simulink model "opdracht1"  (Simulink 6.6)
settings: Solver=ode45  StartTime=0.0  StopTime=inf  RelTol=1e-3
libraries: dspsrcs4 x1, simulink x1, simulink_extras x1
settings Model: Creator=student  LastModifiedBy=student

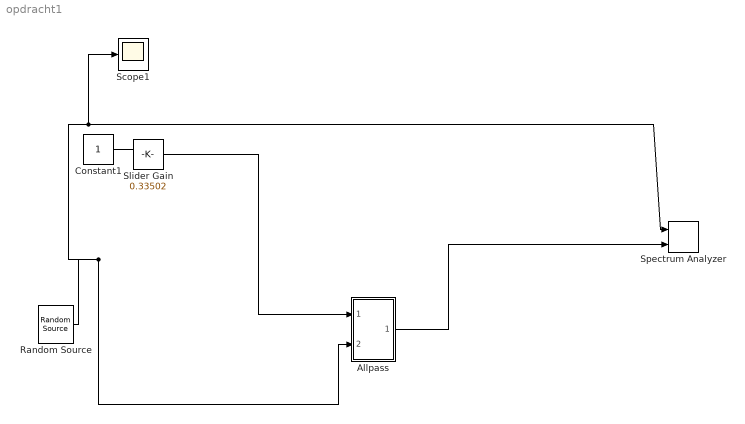
== system opdracht1 ==
  Allpass : Subsystem
  Constant1 : Constant
  Random Source : dspsrcs4/Random Source  SrcType=Uniform  NormMethod=Ziggurat  CltLength=12  MinVal=-10  MaxVal=10  MeanVal=0  VarVal=1  RepMode=Not repeatable  rawSeed=1  IsInherit=off  SampMode=Discrete  SampTime=1  SampFrame=1  DataType=Double  OutComplex=Real
  Scope1 : Scope
  Slider Gain : simulink/Math Operations/Slider Gain  SystemSampleTime=-1  low=0  gain=0.33502  high=1
  Spectrum Analyzer : simulink_extras/Additional Sinks/Spectrum Analyzer  SystemSampleTime=-1  npts=1024  fftpts=1024  HowOften=64  sampleT=1
  wires:
  Random Source/1 -> Scope1/1, Spectrum Analyzer/1, Allpass/2(In2)
  Constant1/1 -> Slider Gain/1
  Slider Gain/1 -> Allpass/1(In1)
  Allpass/1(Out1) -> Spectrum Analyzer/2

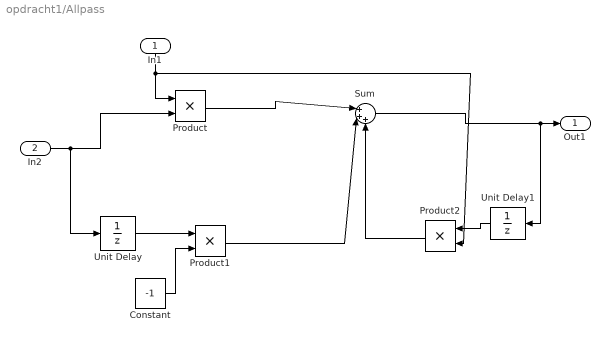
== system opdracht1/Allpass ==
  In1 : Inport  Orientation=down
  In2 : Inport  Port=2
  Constant : Constant  Value=-1
  Product : Product  RndMeth=Zero
  Product1 : Product  RndMeth=Zero
  Product2 : Product  Orientation=left  RndMeth=Zero
  Sum : Sum  Inputs=|+++
  Unit Delay : UnitDelay
  Unit Delay1 : UnitDelay  Orientation=left
  Out1 : Outport
  wires:
  Product/1 -> Sum/1
  Product1/1 -> Sum/2
  In1/1 -> Product2/2, Product/1
  Unit Delay/1 -> Product1/1
  Constant/1 -> Product1/2
  Unit Delay1/1 -> Product2/1
  Product2/1 -> Sum/3
  Sum/1 -> Unit Delay1/1, Out1/1
  In2/1 -> Product/2, Unit Delay/1
